simulink model "simulation_motor"  (R2018a)
settings: Solver=FixedStepAuto  StartTime=0.0  StopTime=10.0  FixedStep=0.001  RelTol=1e-3
settings Model: Creator=ayush2  LastModifiedBy=ayush2

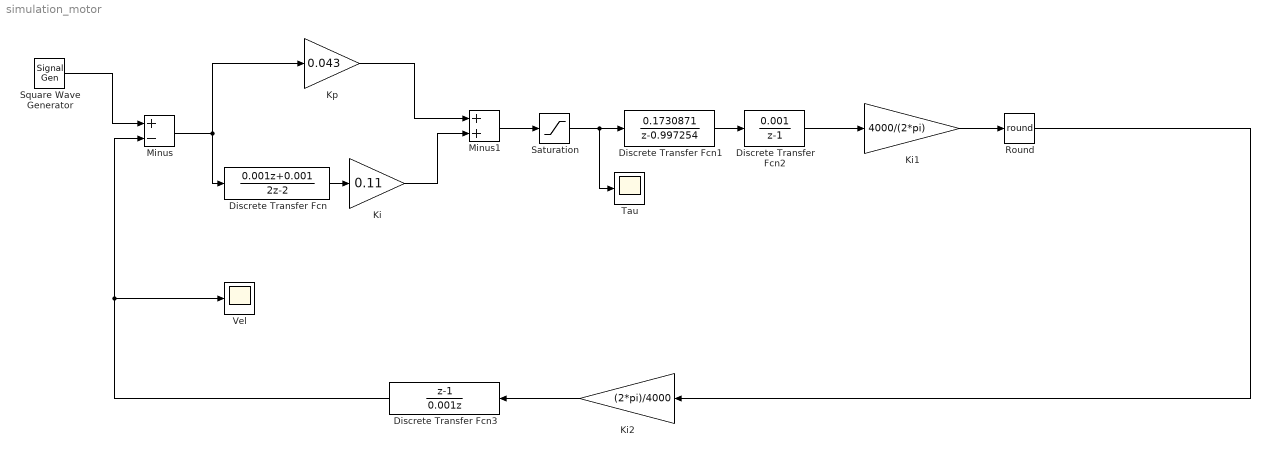
== system simulation_motor ==
  Discrete Transfer Fcn : DiscreteTransferFcn  Numerator=[0.001 0.001]  Denominator=[2 -2]
  Discrete Transfer Fcn1 : DiscreteTransferFcn  Numerator=[0.1730871]  Denominator=[1 -0.997254]
  Discrete Transfer Fcn2 : DiscreteTransferFcn  Numerator=[0.001]  Denominator=[1 -1]
  Discrete Transfer Fcn3 : DiscreteTransferFcn  Numerator=[1 -1]  Denominator=[0.001 0]
  Ki : Gain  Gain=0.11
  Ki1 : Gain  Gain=4000/(2*pi)
  Ki2 : Gain  Gain=(2*pi)/4000
  Kp : Gain  Gain=0.043
  Minus : Sum  Inputs=+-
  Minus1 : Sum
  Round : Rounding  Operator=round
  Saturation : Saturate  UpperLimit=10  LowerLimit=-10
  Square Wave Generator : SignalGenerator  WaveForm=square  Amplitude=100  Frequency=0.25
  Tau : Scope
  Vel : Scope
  wires:
  Square Wave Generator/1 -> Minus/1
  Minus/1 -> Discrete Transfer Fcn/1, Kp/1
  Discrete Transfer Fcn/1 -> Ki/1
  Kp/1 -> Minus1/1
  Ki/1 -> Minus1/2
  Minus1/1 -> Saturation/1
  Saturation/1 -> Tau/1, Discrete Transfer Fcn1/1
  Discrete Transfer Fcn1/1 -> Discrete Transfer Fcn2/1
  Discrete Transfer Fcn2/1 -> Ki1/1
  Ki1/1 -> Round/1
  Round/1 -> Ki2/1
  Ki2/1 -> Discrete Transfer Fcn3/1
  Discrete Transfer Fcn3/1 -> Vel/1, Minus/2
